simulink model "naive_mel+wifi"  (R2023b)
settings: Solver=ode3  StartTime=0.0  StopTime=inf  RelTol=1e-3  EnableMultiTasking=on
undefined symbols (not defined in the file): hw
libraries: raspberrypiAVlib x2, matrix_library x2, etargetslib x1, audiofeatures x1, raspberrypiNetworklib x1
settings Model: FPTRunName=Active  PacingRate=0.500000  ExtModeTrigDuration=2  Creator=Missy  LastModifiedBy=Missy
settings SolverCC: AlgebraicLoopSolver=TrustRegion  PositivePriorityOrder=on
settings DataIOCC: LimitDataPoints=on  SaveFormat=Array
settings OptimizationCC: EnhancedBackFolding=on  PassReuseOutputArgsAs=Individual arguments  ExpressionDepthLimit=2147483647  ZeroExternalMemoryAtStartup=off  ZeroInternalMemoryAtStartup=off  MaxStackSize=64  OptimizeBlockOrder=speed  DifferentSizesBufferReuse=on  OptimizationCustomize=off  EfficientTunableParamExpr=on
settings DebuggingCC: UnderspecifiedInitializationDetection=Classic  MergeDetectMultiDrivingBlocksExec=none  ParameterTunabilityLossMsg=error  FcnCallInpInsideContextMsg=warning  UnconnectedInputMsg=warning  UnconnectedOutputMsg=warning  UnconnectedLineMsg=warning  AllowSymbolicDim=off  StateNameClashWarn=warning  SubsystemReferenceDiagnosticForUnitTest=warning  SFUnexpectedBacktrackingDiag=warning  SFNoUnconditionalDefaultTransitionDiag=warning  SFExecutionAtInitializationDiag=none  ArithmeticOperatorsInVariantConditions=warning
settings HardwareCC: ProdBitPerLong=64  ProdLargestAtomicInteger=LongLong  ProdLargestAtomicFloat=Double  ProdLongLongMode=on  ProdHWDeviceType=ARM Compatible->ARM 64-bit (LP64)
settings ModelReferenceCC: EnableRefExpFcnMdlSchedulingChecks=on  PropagateSignalLabelsOutOfModel=off
settings SFSimCC: SimUseLocalCustomCode=off  CustomCodeUndefinedFunction=UseInterfaceOnly
settings RTWCC: Description=Embedded Coder  SystemTargetFile=ert.tlc  HardwareBoard=Raspberry Pi (64bit)  TLCOptions="-aInlineSetEventsForThisBaseRateFcn=TLC_FALSE -aSuppressMultiTaskScheduler=TLC_FALSE  -aRateBasedStepFcn=0"  TemplateMakefile=ert_default_tmf  GenerateReport=on  RTWVerbose=off  RTWUseLocalCustomCode=off  Toolchain=GNU GCC Embedded Linux  BuildConfiguration=Faster Runs  LaunchReport=on
settings CodeAppCC: ForceParamTrailComments=on  IgnoreCustomStorageClasses=off  OperatorAnnotations=on  SimulinkDataObjDesc=on  SFDataObjDesc=on  InsertBlockDesc=on
settings ERTTargetCC: SupportVariableSizeSignals=on  ExtModeTransport=2  ExtModeStaticAlloc=on  ExtModeMexFile=ext_xcp  ExtModeIntrfLevel=Level2 - Open
settings ConfigComp: CovMetricSettings=dw  CovSaveCumulativeToWorkspaceVar=on  CovSaveSingleToWorkspaceVar=on  CovExternalEMLEnable=off  CovSFcnEnable=off

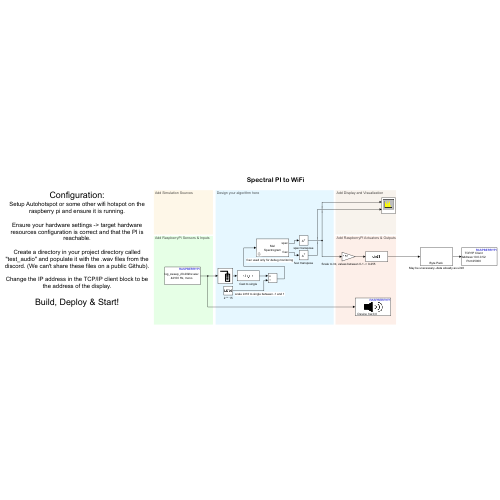
[thumbnail: Simulink's stored preview of the top-level diagram]
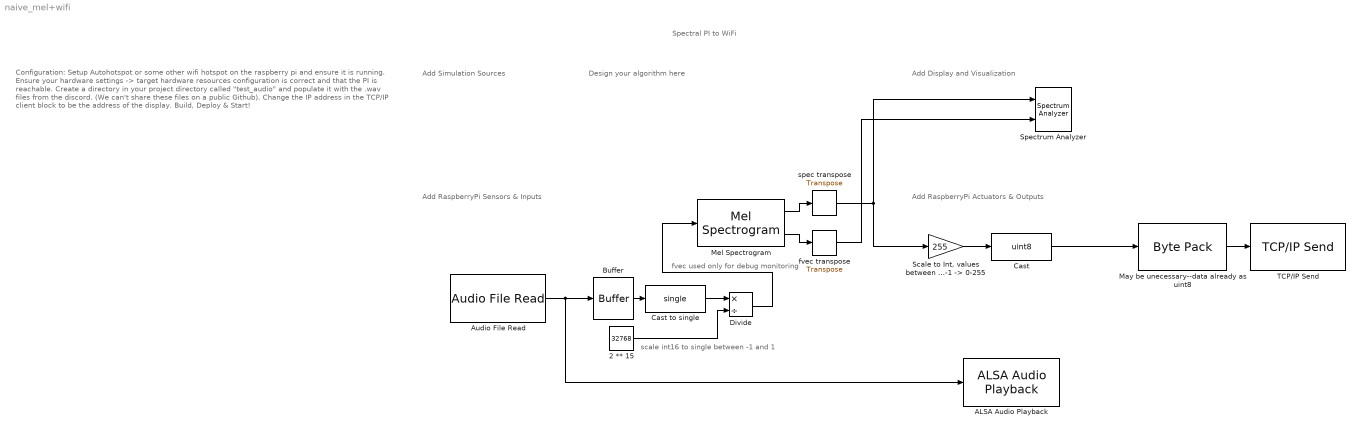
== system naive_mel+wifi ==
  note: Configuration:
      | Setup Autohotspot or some other wifi hotspot on the raspberry pi and ensure it is running.
      |
      | Ensure your hardware settings -> target hardware resources configuration is correct and that the PI is reachable.
      |
      | Create a directory in your project directory called
      | "test_audio" and populate it with the .wav files from the discord. (We can't share these files on a public Github).
      |
      | Change the IP address in the TCP/IP client block to be the address of the display.
      |
      | Build, Deploy & Start!
  note: fvec used only for debug monitoring
  note: scale int16 to single between -1 and 1
  note: Add Simulation Sources
  note: Add Display and Visualization
  note: Design your algorithm here
  note: Add RaspberryPi Actuators & Outputs
  note: Spectral PI to WiFi
  note: Add RaspberryPi Sensors & Inputs
  2 ** 15 : Constant  Value=32768
  ALSA Audio Playback : raspberrypiAVlib/ALSA Audio Playback  deviceStr=hw:0,0  sampleRateEnum=44100  queueDuration=0.5  blockPlatform=LINUX
  Audio File Read : raspberrypiAVlib/Audio File Read  FileName=C:\spectral_art\test_audio\log_sweep_20-20khz.wav  PlayCount=Inf  OutputEOFIndicator=off  SamplesPerFrame=4410
  Buffer : Buffer  N=1024  OutputFrames=off
  Cast : DataTypeConversion  OutDataTypeStr=uint8  RndMeth=Nearest
  Cast to single : DataTypeConversion  OutDataTypeStr=single  SaturateOnIntegerOverflow=off  RndMeth=Floor
  Divide : Product  Inputs=*/
  May be unecessary--data already as uint8 : etargetslib/Byte Pack  datatypes={['uint8']}  byteAlign=1
  Mel Spectrogram : audiofeatures/Mel Spectrogram  FrequencyScale=mel  AutoNumBands=off  NumBands=8  AutoFrequencyRange=on  FrequencyRange=[0, 22050]  FilterBankDesignDomain=warped  FilterBankNormalization=none  MelStyle=oshaughnessy  OutputFrequencyVector=on  WindowParameter=hamming(1024,'periodic')  WindowNormalization=on  OverlapLength=512  AutoFFTLength=on  FFTLength=1024  SpectrumType=magnitude  NumHops=1  NumHopsOverlap=0  InheritSampleRate=off  SampleRate=44.1e3
  "Scale to Int, values between 0-1 -> 0-255" : Gain  Gain=255
  Spectrum Analyzer : SpectrumAnalyzer  NumInputPorts=2  WindowPosition=[1.000000,49.000000,1280.000000,649.000000,]  ScopeFrameLocation=window  InputDomain=Frequency  SampleRateSource=Property  SampleRate=44.1e3  PlotAsTwoSidedSpectrum=off  FrequencyScale=Log  AxesScaling=Manual  FrequencySpan=Start and stop frequencies  StartFrequency=20  StopFrequency=20e3  FrequencyVectorSource=Input port  SpectrumUnits=Auto  YLimits=[0,5]  ColorLimits=[-16.26031024,115.75673353]
  TCP/IP Send : raspberrypiNetworklib/TCP//IP Send  Mode_=Client  LocalServerPort_=25000  RemoteAddr_=10.0.0.52  RemoteServerPort_=25000  SimulateUsing=Code generation  ClientPortBindingSelection_=off  ClientPortToBind_=35000  BlockingMode_=off  BlockTimeout_=0.1  BlockPlatform=RASPBERRYPI
  fvec transpose : matrix_library/Transpose
  spec transpose : matrix_library/Transpose
  wires:
  Audio File Read/1 -> ALSA Audio Playback/1, Buffer/1
  spec transpose/1 -> "Scale to Int, values between 0-1 -> 0-255"/1, Spectrum Analyzer/1
  Mel Spectrogram/1 -> spec transpose/1
  Mel Spectrogram/2 -> fvec transpose/1
  fvec transpose/1 -> Spectrum Analyzer/2
  May be unecessary--data already as uint8/1 -> TCP/IP Send/1
  Cast/1 -> May be unecessary--data already as uint8/1
  2 ** 15/1 -> Divide/2
  Buffer/1 -> Cast to single/1
  Divide/1 -> Mel Spectrogram/1
  Cast to single/1 -> Divide/1
  "Scale to Int, values between 0-1 -> 0-255"/1 -> Cast/1
